simulink model "DataPath"  (R2025a)
settings: Solver=FixedStepAuto  StartTime=0  StopTime=0.02  FixedStep=1e-7  RelTol=1e-3
undefined symbols (not defined in the file): Bit_1, Bit_2, Bit_3, Bit_4, Bit_5, Bit_6, Bit_7, Bit_8
libraries: simulink_extras x126, fl_lib x34, nesl_utility x18, simulink x2
(part 3 of 7)

== system DataPath/Subsystem1/Normalize Div ==
  Enable : Inport
  Step Bus : Inport  Port=2
  MSB : Inport  Port=3
  Eval-ICS : Inport  Port=4
  Store B1-ICS : Inport  Port=5
  Zero : Inport  Port=6
  AND{2..8,10..11} (9 alike) : Logic  IconShape=distinctive  AllPortsSameDT=off  OutDataTypeStr=boolean
  D Latch : simulink_extras/Flip Flops/D Latch
  Demux : Demux  Outputs=5
  OR{,5..7} (4 alike) : Logic  Operator=OR  IconShape=distinctive  AllPortsSameDT=off  OutDataTypeStr=boolean
  S-R Flip-Flop1 : simulink_extras/Flip Flops/S-R Flip-Flop  initial_condition=0
  S-R Flip-Flop2 : simulink_extras/Flip Flops/S-R Flip-Flop  initial_condition=0
  Subsystem1 : Subsystem
  Subsystem8 : Subsystem
  Out ALU : Outport
  Out A1 : Outport  Port=2
  Out B1 : Outport  Port=3
  Store A1 : Outport  Port=4
  Store B1 : Outport  Port=5
  NegA : Outport  Port=6
  ADD : Outport  Port=7
  MSB x : Outport  Port=8
  MSB y : Outport  Port=9
  END-ND : Outport  Port=10
  Div/0 : Outport  Port=11
  wires:
  S-R Flip-Flop1/1 -> AND7/2, OR5/1
  Enable/1 -> AND6/1, AND5/1, AND4/1, AND3/1, AND2/1
  AND2/1 -> OR6/1, D Latch/2
  Subsystem8/2(Q) -> MSB x/1, AND7/1
  S-R Flip-Flop2/1 -> OR6/2, AND8/2, OR5/2
  Subsystem1/2(Q) -> MSB y/1, AND8/1
  AND3/1 -> AND11/1, AND10/1
  AND10/1 -> Div/0/1
  AND5/1 -> S-R Flip-Flop2/1
  MSB/1 -> Subsystem1/1(Data), Subsystem8/1(Data)
  D Latch/2 -> AND11/2
  AND6/1 -> OR7/2, S-R Flip-Flop2/2, END-ND/1
  AND4/1 -> OR7/1
  D Latch/1 -> AND10/2
  Zero/1 -> D Latch/1
  OR7/1 -> S-R Flip-Flop1/2
  Eval-ICS/1 -> Subsystem1/2(CLK)
  OR5/1 -> Out ALU/1
  Store B1-ICS/1 -> Subsystem8/2(CLK)
  OR6/1 -> OR/2
  AND11/1 -> S-R Flip-Flop1/1
  Step Bus/1 -> Demux/1
  Demux/4 -> AND5/2
  Demux/3 -> AND4/2
  Demux/2 -> AND3/2
  Demux/1 -> AND2/2
  Demux/5 -> AND6/2
  AND7/1 -> Store A1/1, Out A1/1, ADD/1, NegA/1
  AND8/1 -> OR/1, Store B1/1
  OR/1 -> Out B1/1

== system DataPath/Subsystem1/SCS ==
  CLR : Inport
  Multiplying : Inport  Port=2
  Dividing : Inport  Port=3
  Evaluating : Inport  Port=4
  Output DP-Mult : Inport  Port=5
  Output DP-Div : Inport  Port=6
  CLK : Inport  Port=7
  END-CD : Inport  Port=8
  END-ND : Inport  Port=9
  DIV/0 : Inport  Port=10
  AND{,1..4} (5 alike) : Logic  IconShape=distinctive  AllPortsSameDT=off  OutDataTypeStr=boolean
  Delay One Step : Delay  DelayLength=1  SampleTime=1e-6
  Delay One Step1 : Delay  DelayLength=1  SampleTime=1e-6
  Delay One Step{2,4..7} (5 alike) : Delay  DelayLength=1
  OR4 : Logic  Operator=OR  Inputs=3  IconShape=distinctive  AllPortsSameDT=off  OutDataTypeStr=boolean
  OR5 : Logic  Operator=OR  IconShape=distinctive  AllPortsSameDT=off  OutDataTypeStr=boolean
  Rate Transition : RateTransition
  Rate Transition1 : RateTransition
  S-R Flip-Flop : simulink_extras/Flip Flops/S-R Flip-Flop  initial_condition=0
  S-R Flip-Flop1 : simulink_extras/Flip Flops/S-R Flip-Flop  initial_condition=0
  S-R Flip-Flop2 : simulink_extras/Flip Flops/S-R Flip-Flop  initial_condition=0
  Enable Stepper : Outport
  CCLK : Outport  Port=2
  Enable-Mult : Outport  Port=3
  Enable-CD : Outport  Port=4
  Enable-ND : Outport  Port=5
  Enable-SDR : Outport  Port=6
  wires:
  CLR/1 -> S-R Flip-Flop2/2, S-R Flip-Flop1/2, Rate Transition1/1
  Output DP-Div/1 -> OR4/2
  DIV/0/1 -> OR4/3
  Output DP-Mult/1 -> OR4/1
  Multiplying/1 -> AND/2
  Dividing/1 -> AND2/1
  Evaluating/1 -> AND2/2, AND/1
  S-R Flip-Flop2/2 -> AND4/2
  END-ND/1 -> Delay One Step1/1
  END-CD/1 -> Delay One Step/1
  OR4/1 -> Delay One Step7/1
  AND2/1 -> OR5/1, AND3/1
  AND/1 -> OR5/2, Delay One Step5/1
  S-R Flip-Flop1/1 -> AND4/1
  S-R Flip-Flop1/2 -> AND3/2
  CLK/1 -> AND1/1
  S-R Flip-Flop/1 -> Delay One Step6/1
  OR5/1 -> Enable Stepper/1
  AND3/1 -> Delay One Step2/1
  AND4/1 -> Rate Transition/1
  AND1/1 -> CCLK/1
  S-R Flip-Flop2/1 -> Delay One Step4/1
  Delay One Step2/1 -> Enable-ND/1
  Rate Transition/1 -> Enable-CD/1
  Delay One Step4/1 -> Enable-SDR/1
  Delay One Step5/1 -> Enable-Mult/1
  Delay One Step/1 -> S-R Flip-Flop2/1
  Delay One Step1/1 -> S-R Flip-Flop1/1
  Delay One Step6/1 -> AND1/2
  Delay One Step7/1 -> S-R Flip-Flop/2
  Rate Transition1/1 -> S-R Flip-Flop/1

== system DataPath/Subsystem1/Sign Div result ==
  Enable : Inport
  Step Bus : Inport  Port=2
  MOD : Inport  Port=3
  MSB x : Inport  Port=4
  MSB y : Inport  Port=5
  AND{,1..9} (10 alike) : Logic  IconShape=distinctive  AllPortsSameDT=off  OutDataTypeStr=boolean
  Delay : Delay  DelayLength=1  InputProcessing=Columns as channels (frame based)  SampleTime=1e-6
  Delay1 : Delay  DelayLength=1  InputProcessing=Columns as channels (frame based)  SampleTime=1e-6
  Delay2 : Delay  DelayLength=1  InputProcessing=Columns as channels (frame based)  SampleTime=1e-6
  Demux : Demux  Outputs=5
  OR{,1..3,5,9} (6 alike) : Logic  Operator=OR  IconShape=distinctive  AllPortsSameDT=off  OutDataTypeStr=boolean
  S-R Flip-Flop{,1..3} (4 alike) : simulink_extras/Flip Flops/S-R Flip-Flop  initial_condition=0
  XOR : Logic  Operator=XOR  IconShape=distinctive  AllPortsSameDT=off  OutDataTypeStr=boolean
  Out ALU : Outport
  Out A1 : Outport  Port=2
  Out B2 : Outport  Port=3
  Store A1 : Outport  Port=4
  Store B2 : Outport  Port=5
  NegA : Outport  Port=6
  Output DP : Outport  Port=7
  ADD : Outport  Port=8
  wires:
  Enable/1 -> AND6/1, AND5/1, AND4/1, AND3/1, AND2/1
  Step Bus/1 -> Demux/1
  Demux/4 -> S-R Flip-Flop3/2, AND5/2
  Demux/3 -> AND4/2
  Demux/2 -> AND3/2
  Demux/1 -> AND2/2, Delay1/1
  Demux/5 -> AND6/2
  MSB y/1 -> XOR/2
  MSB x/1 -> AND7/1, XOR/1
  AND2/1 -> S-R Flip-Flop/1
  OR9/1 -> S-R Flip-Flop/2
  AND3/1 -> Delay2/1, OR9/1
  AND6/1 -> OR2/2, OR9/2, AND9/1, AND/1, AND8/1
  S-R Flip-Flop/1 -> AND1/2
  XOR/1 -> AND1/1
  OR1/1 -> OR5/1, Out B2/1
  AND1/1 -> OR1/1, Store B2/1
  OR2/1 -> S-R Flip-Flop1/2
  AND4/1 -> S-R Flip-Flop1/1
  AND5/1 -> OR2/1
  S-R Flip-Flop1/1 -> AND7/2
  OR3/1 -> OR5/2, Out A1/1
  AND7/1 -> OR/1, OR3/1, Store A1/1, NegA/1
  S-R Flip-Flop3/1 -> AND8/2
  AND/1 -> OR1/2
  AND8/1 -> OR3/2
  OR5/1 -> Out ALU/1
  AND9/1 -> Output DP/1, OR/2
  S-R Flip-Flop2/1 -> Delay/1
  OR/1 -> ADD/1
  MOD/1 -> S-R Flip-Flop3/1
  S-R Flip-Flop3/2 -> AND/2
  Delay/1 -> AND9/2
  Delay1/1 -> S-R Flip-Flop2/2
  Delay2/1 -> S-R Flip-Flop2/1

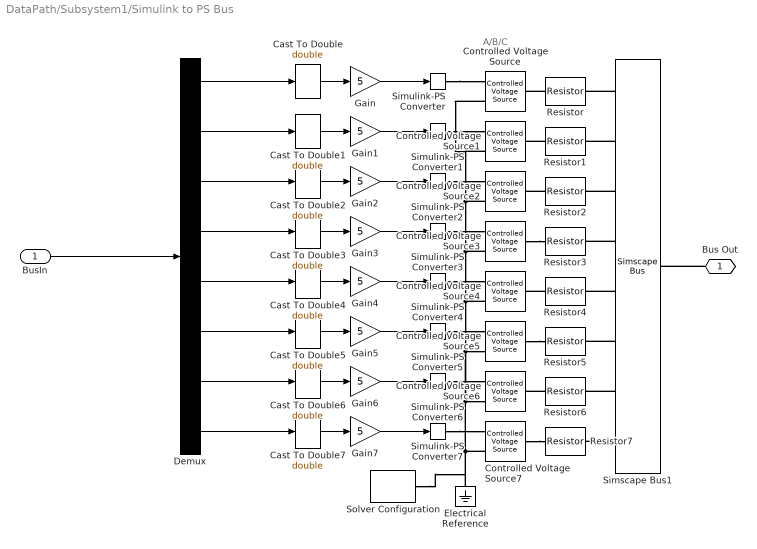
== system DataPath/Subsystem1/Simulink to PS Bus ==
  note: A/B/C
  BusIn : Inport
  Cast To Double{,1..7} (8 alike) : DataTypeConversion  OutDataTypeStr=double  SaturateOnIntegerOverflow=off  RndMeth=Floor
  Controlled Voltage Source{,1..7} (8 alike) : fl_lib/Electrical/Electrical Sources/Controlled Voltage Source
  Demux : Demux  Outputs=8
  Electrical Reference : fl_lib/Electrical/Electrical Elements/Electrical Reference
  Gain{,1..7} (8 alike) : Gain  Gain=5
  Resistor{,1..7} (8 alike) : fl_lib/Electrical/Electrical Elements/Resistor  R=1 Ohm  i_specify=off  i_priority=None  i=0 A  i_nominal_specify=off  i_nominal_value=1  i_nominal_unit=A  v_specify=off  v_priority=None  v=0 V  v_nominal_specify=off  v_nominal_value=1  v_nominal_unit=V
  Simscape Bus1 : SimscapeBus  HierarchyStrings=Bit_8;Bit_7;Bit_6;Bit_5;Bit_4;Bit_3;Bit_2;Bit_1
  Simulink-PS Converter{,1..7} (8 alike) : nesl_utility/Simulink-PS Converter  PhysicalDomain=network_engine_domain  SubClassName=ps_input  LeftPortType=input  RightPortType=output  PseudoPeriodic=off  Frequencies=[]  NoiseDistribution=none  NoiseParameters=[]  Unit=1  AffineConversion=off  FilteringAndDerivatives=provide  SimscapeFilterOrder=1  InputFilterTimeConstant=0.001  UdotUserProvided=0
  Solver Configuration : nesl_utility/Solver Configuration  PhysicalDomain=network_engine_domain  SubClassName=solver  LeftPortType=input  RightPortType=generic  Tones=[]  Harmonics=[]  SimulateNoise=off  Profile=off  UseLocalSampling=off  EnableSwitchedLinearOptims=on  FrequencyDomain=off  UseCCode=off  RelTol=0.001  AbsTol=0.001  MinStep=1e-09  ToWorkspace=off  RevertToSquareIcSolve=off  NumHomotopyIterations=100  PhasorMode=off  PhasorModeNumHarmonics=1  ConsistencySolver=NEWTON_XTOL_AFTER_FTOL  IndexReductionMethod=DerivativeReplacement  DoDC=off  ResidualTolerance=1e-09  ConsistencyTolSource=GLOBAL  ConsistencyAbsTol=0.001  ConsistencyRelTol=0.001  ConsistencyTolFactor=0.001  UseLocalSolver=off  LocalSolverChoice=NE_BACKWARD_EULER_ADVANCER  ResolveIndetEquations=on  FunctionEvalNumThread=1  LocalSolverSampleTime=0.001  DoFixedCost=off  MaxNonlinIter=3  MaxModeIter=2  ComputeImpulses=off  ImpulseIterations=2  LinearAlgebra=auto  LinearAlgebraNumThread=0  EquationFormulation=NE_TIME_EF  DelaysMemoryBudget=1024  AutomaticFiltering=on  FilteringTimeConstant=0.001  PartitionStorageMethod=AS_NEEDED  PartitionMemoryBudget=1024  PartitionMethod=ROBUST  MultibodyUseLocalSolver=off  MultibodyLocalSolverChoice=ODE1  MultibodyLocalSolverSampleTime=0.001
  Bus Out : PMIOPort  Side=Right
  wires:
  BusIn/1 -> Demux/1
  Demux/5 -> Cast To Double4/1
  Cast To Double5/1 -> Gain5/1
  Cast To Double6/1 -> Gain6/1
  Cast To Double7/1 -> Gain7/1
  Gain/1 -> Simulink-PS Converter/1
  Demux/2 -> Cast To Double1/1
  Demux/4 -> Cast To Double3/1
  Gain5/1 -> Simulink-PS Converter5/1
  Gain4/1 -> Simulink-PS Converter4/1
  Gain2/1 -> Simulink-PS Converter2/1
  Cast To Double2/1 -> Gain2/1
  Cast To Double4/1 -> Gain4/1
  Gain6/1 -> Simulink-PS Converter6/1
  Cast To Double3/1 -> Gain3/1
  Cast To Double/1 -> Gain/1
  Cast To Double1/1 -> Gain1/1
  Demux/7 -> Cast To Double6/1
  Demux/1 -> Cast To Double/1
  Gain3/1 -> Simulink-PS Converter3/1
  Demux/6 -> Cast To Double5/1
  Gain7/1 -> Simulink-PS Converter7/1
  Demux/8 -> Cast To Double7/1
  Demux/3 -> Cast To Double2/1
  Gain1/1 -> Simulink-PS Converter1/1
  connections:
  Controlled Voltage Source2/RConn2 -- Controlled Voltage Source/RConn2 -- Controlled Voltage Source1/RConn2 -- Controlled Voltage Source3/RConn2 -- Controlled Voltage Source4/RConn2 -- Controlled Voltage Source5/RConn2 -- Controlled Voltage Source6/RConn2 -- Controlled Voltage Source7/RConn2 -- Solver Configuration/RConn1 -- Electrical Reference/LConn1
  Simscape Bus1/LConn7 -- Resistor6/RConn1
  Simscape Bus1/LConn5 -- Resistor4/RConn1
  Simscape Bus1/LConn8 -- Resistor7/RConn1
  Simulink-PS Converter5/RConn1 -- Controlled Voltage Source5/RConn1
  Simulink-PS Converter4/RConn1 -- Controlled Voltage Source4/RConn1
  Simulink-PS Converter6/RConn1 -- Controlled Voltage Source6/RConn1
  Simulink-PS Converter/RConn1 -- Controlled Voltage Source/RConn1
  Simulink-PS Converter1/RConn1 -- Controlled Voltage Source1/RConn1
  Simscape Bus1/LConn4 -- Resistor3/RConn1
  Controlled Voltage Source5/LConn1 -- Resistor5/LConn1
  Simulink-PS Converter7/RConn1 -- Controlled Voltage Source7/RConn1
  Simulink-PS Converter3/RConn1 -- Controlled Voltage Source3/RConn1
  Simscape Bus1/LConn2 -- Resistor1/RConn1
  Simulink-PS Converter2/RConn1 -- Controlled Voltage Source2/RConn1
  Resistor2/LConn1 -- Controlled Voltage Source2/LConn1
  Resistor/LConn1 -- Controlled Voltage Source/LConn1
  Simscape Bus1/LConn1 -- Resistor/RConn1
  Resistor1/LConn1 -- Controlled Voltage Source1/LConn1
  Simscape Bus1/LConn3 -- Resistor2/RConn1
  Controlled Voltage Source3/LConn1 -- Resistor3/LConn1
  Resistor4/LConn1 -- Controlled Voltage Source4/LConn1
  Simscape Bus1/LConn6 -- Resistor5/RConn1
  Resistor6/LConn1 -- Controlled Voltage Source6/LConn1
  Controlled Voltage Source7/LConn1 -- Resistor7/LConn1
  Bus Out/RConn1 -- Simscape Bus1/RConn1

== system DataPath/Subsystem1/Stepper ==
  Reset : Inport
  Enable : Inport  Port=2
  CLK : Inport  Port=3
  Subsystem1 : Subsystem
      settings: PortSchema="{\"entries\":[{\"content\":{\"sides\":[{\"content\":{\"connectorIds\":[\"In1\",\"Out3\",\"In2\"]},\"type\":\"ConnectorPlacement.EquallySpacedRectSide\",\"uuid\":\"a2ffd4d4-cb1e-427b-87da-e82cfc528a9f\"},{\"content\":{\"connectorIds\":[\"Out1\",\"In3\",\"Out2\"],\"side\":\"RIGHT\"},\"type\":\"ConnectorPlacement.EquallySpacedRectSide\",\"uuid\":\"71314638-bff7-4a07-ab36-c1b86a64e6a5\"},{\"content\":{\"side\":\"TOP\"},\"type\":\"ConnectorPlacement.EquallySpacedRectSide\",\"uuid\":\"4ed90d18-bd24-4652-9ebf-70eb68655746\"},{\"content\":{\"side\":\"BOTTOM\"},\"type\":\"ConnectorPlacement.EquallySpacedRectSide\",\"uuid\":\"b13ca18e-58ec-4b33-9e47-5b828845d5a6\"}]},\"type\":\"ConnectorPlacement.EquallySpacedConnector\",\"uuid\":\"af20c32a-17bf-45dc-90e2-7848574669b1\"}],\"packageUris\":[\"http://schema.mathworks.com/mf0/Connector/R2020b\"],\"version\":\"1.0\"}"
  Subsystem2 : Subsystem
      settings: PortSchema="{\"entries\":[{\"content\":{\"sides\":[{\"content\":{\"connectorIds\":[\"In1\",\"Out3\",\"In2\"]},\"type\":\"ConnectorPlacement.EquallySpacedRectSide\",\"uuid\":\"a2ffd4d4-cb1e-427b-87da-e82cfc528a9f\"},{\"content\":{\"connectorIds\":[\"Out1\",\"In3\",\"Out2\"],\"side\":\"RIGHT\"},\"type\":\"ConnectorPlacement.EquallySpacedRectSide\",\"uuid\":\"71314638-bff7-4a07-ab36-c1b86a64e6a5\"},{\"content\":{\"side\":\"TOP\"},\"type\":\"ConnectorPlacement.EquallySpacedRectSide\",\"uuid\":\"4ed90d18-bd24-4652-9ebf-70eb68655746\"},{\"content\":{\"side\":\"BOTTOM\"},\"type\":\"ConnectorPlacement.EquallySpacedRectSide\",\"uuid\":\"b13ca18e-58ec-4b33-9e47-5b828845d5a6\"}]},\"type\":\"ConnectorPlacement.EquallySpacedConnector\",\"uuid\":\"af20c32a-17bf-45dc-90e2-7848574669b1\"}],\"packageUris\":[\"http://schema.mathworks.com/mf0/Connector/R2020b\"],\"version\":\"1.0\"}"
  Subsystem3 : Subsystem
      settings: PortSchema="{\"entries\":[{\"content\":{\"sides\":[{\"content\":{\"connectorIds\":[\"In1\",\"Out3\",\"In2\"]},\"type\":\"ConnectorPlacement.EquallySpacedRectSide\",\"uuid\":\"a2ffd4d4-cb1e-427b-87da-e82cfc528a9f\"},{\"content\":{\"connectorIds\":[\"Out1\",\"In3\",\"Out2\"],\"side\":\"RIGHT\"},\"type\":\"ConnectorPlacement.EquallySpacedRectSide\",\"uuid\":\"71314638-bff7-4a07-ab36-c1b86a64e6a5\"},{\"content\":{\"side\":\"TOP\"},\"type\":\"ConnectorPlacement.EquallySpacedRectSide\",\"uuid\":\"4ed90d18-bd24-4652-9ebf-70eb68655746\"},{\"content\":{\"side\":\"BOTTOM\"},\"type\":\"ConnectorPlacement.EquallySpacedRectSide\",\"uuid\":\"b13ca18e-58ec-4b33-9e47-5b828845d5a6\"}]},\"type\":\"ConnectorPlacement.EquallySpacedConnector\",\"uuid\":\"af20c32a-17bf-45dc-90e2-7848574669b1\"}],\"packageUris\":[\"http://schema.mathworks.com/mf0/Connector/R2020b\"],\"version\":\"1.0\"}"
  Subsystem4 : Subsystem
      settings: PortSchema="{\"entries\":[{\"content\":{\"sides\":[{\"content\":{\"connectorIds\":[\"In1\",\"Out3\",\"In2\"]},\"type\":\"ConnectorPlacement.EquallySpacedRectSide\",\"uuid\":\"a2ffd4d4-cb1e-427b-87da-e82cfc528a9f\"},{\"content\":{\"connectorIds\":[\"Out1\",\"In3\",\"Out2\"],\"side\":\"RIGHT\"},\"type\":\"ConnectorPlacement.EquallySpacedRectSide\",\"uuid\":\"71314638-bff7-4a07-ab36-c1b86a64e6a5\"},{\"content\":{\"side\":\"TOP\"},\"type\":\"ConnectorPlacement.EquallySpacedRectSide\",\"uuid\":\"4ed90d18-bd24-4652-9ebf-70eb68655746\"},{\"content\":{\"side\":\"BOTTOM\"},\"type\":\"ConnectorPlacement.EquallySpacedRectSide\",\"uuid\":\"b13ca18e-58ec-4b33-9e47-5b828845d5a6\"}]},\"type\":\"ConnectorPlacement.EquallySpacedConnector\",\"uuid\":\"af20c32a-17bf-45dc-90e2-7848574669b1\"}],\"packageUris\":[\"http://schema.mathworks.com/mf0/Connector/R2020b\"],\"version\":\"1.0\"}"
  Step 0 : Outport
  Step 1 : Outport  Port=2
  Step 2 : Outport  Port=3
  Step 3 : Outport  Port=4
  Step 4 : Outport  Port=5
  wires:
  CLK/1 -> Subsystem1/2(CLK), Subsystem4/2(CLK), Subsystem3/2(CLK), Subsystem2/2(CLK)
  Subsystem4/1("Step_{n}") -> Step 4/1
  Reset/1 -> Subsystem4/3("OR_{n+1}")
  Enable/1 -> Subsystem2/1("Step_{n-1}")
  Subsystem2/1("Step_{n}") -> Subsystem1/1("Step_{n-1}"), Step 1/1
  Subsystem1/3("OR_{n}") -> Subsystem2/3("OR_{n+1}")
  Subsystem1/1("Step_{n}") -> Subsystem3/1("Step_{n-1}"), Step 2/1
  Subsystem3/3("OR_{n}") -> Subsystem1/3("OR_{n+1}")
  Subsystem3/1("Step_{n}") -> Subsystem4/1("Step_{n-1}"), Step 3/1
  Subsystem4/3("OR_{n}") -> Subsystem3/3("OR_{n+1}")
  Subsystem2/2("!Step_{n}") -> Step 0/1

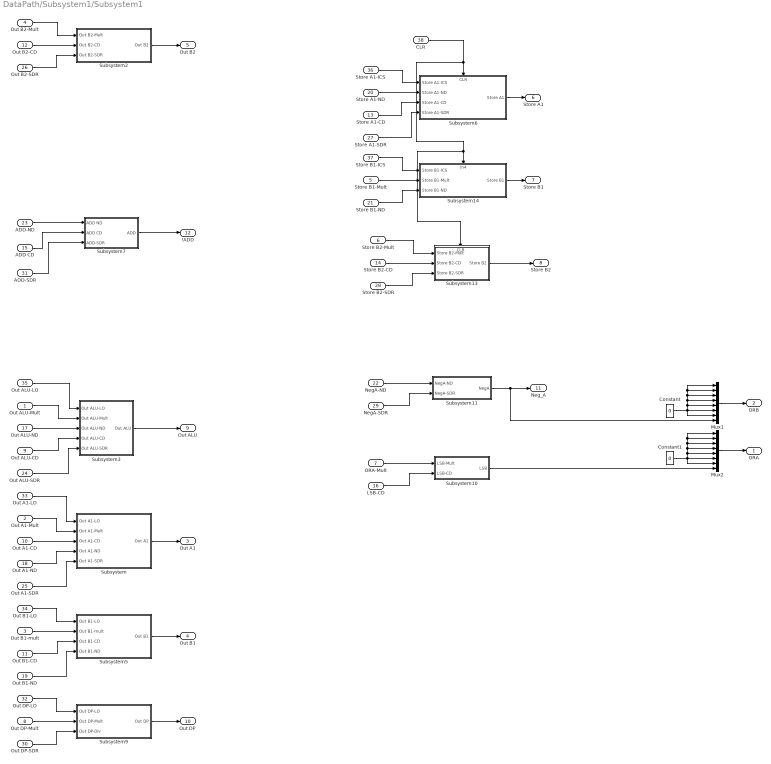
== system DataPath/Subsystem1/Subsystem1 ==
  Out ALU-Mult : Inport
  Out A1-Mult : Inport  Port=2
  Out B1-mult : Inport  Port=3
  Out B2-Mult : Inport  Port=4
  Store B1-Mult : Inport  Port=5
  Store B2-Mult : Inport  Port=6
  ORA-Mult : Inport  Port=7
  Out DP-Mult : Inport  Port=8
  Out ALU-CD : Inport  Port=9
  Out A1-CD : Inport  Port=10
  Out B1-CD : Inport  Port=11
  Out B2-CD : Inport  Port=12
  Store A1-CD : Inport  Port=13
  Store B2-CD : Inport  Port=14
  ADD CD : Inport  Port=15
  LSB-CD : Inport  Port=16
  Out ALU-ND : Inport  Port=17
  Out A1-ND : Inport  Port=18
  Out B1-ND : Inport  Port=19
  Store A1-ND : Inport  Port=20
  Store B1-ND : Inport  Port=21
  NegA-ND : Inport  Port=22
  ADD-ND : Inport  Port=23
  Out ALU-SDR : Inport  Port=24
  Out A1-SDR : Inport  Port=25
  Out B2-SDR : Inport  Port=26
  Store A1-SDR : Inport  Port=27
  Store B2-SDR : Inport  Port=28
  NegA-SDR : Inport  Port=29
  Out DP-SDR : Inport  Port=30
  ADD-SDR : Inport  Port=31
  Out DP-LO : Inport  Port=32
  Out A1-LO : Inport  Port=33
  Out B1-LO : Inport  Port=34
  Out ALU-LO : Inport  Port=35
  Store A1-ICS : Inport  Port=36
  Store B1-ICS : Inport  Port=37
  CLR : Inport  Port=38
  Constant : Constant  Value=0  OutDataTypeStr=boolean
  Constant1 : Constant  Value=0  OutDataTypeStr=boolean
  Mux1 : Mux  Inputs=8
  Mux2 : Mux  Inputs=8
  Subsystem : Subsystem
  Subsystem10 : Subsystem
  Subsystem11 : Subsystem
  Subsystem13 : Subsystem
      settings: PortSchema="{\"entries\":[{\"content\":{\"sides\":[{\"content\":{\"connectorIds\":[\"In1\",\"In2\",\"In3\"]},\"type\":\"ConnectorPlacement.EquallySpacedRectSide\",\"uuid\":\"2d56d23b-6617-4046-a99f-24fef166ef06\"},{\"content\":{\"connectorIds\":[\"Out1\"],\"side\":\"RIGHT\"},\"type\":\"ConnectorPlacement.EquallySpacedRectSide\",\"uuid\":\"3c4df583-b380-4f6c-803a-8385e40aa290\"},{\"content\":{\"connectorIds\":[\"In4\"],\"side\":\"TOP\"},\"type\":\"ConnectorPlacement.EquallySpacedRectSide\",\"uuid\":\"43dc231e-5ab9-4cdd-8239-1dcaab484e6e\"}]},\"type\":\"ConnectorPlacement.EquallySpacedConnector\",\"uuid\":\"3f11ba61-6682-48c0-a60b-53ec54e9a9d7\"}],\"packageUris\":[\"http://schema.mathworks.com/mf0/Connector/R2020b\"],\"version\":\"1.0\"}"
  Subsystem14 : Subsystem
      settings: PortSchema="{\"entries\":[{\"content\":{\"sides\":[{\"content\":{\"connectorIds\":[\"In1\",\"In2\",\"In3\"]},\"type\":\"ConnectorPlacement.EquallySpacedRectSide\",\"uuid\":\"2d56d23b-6617-4046-a99f-24fef166ef06\"},{\"content\":{\"connectorIds\":[\"Out1\"],\"side\":\"RIGHT\"},\"type\":\"ConnectorPlacement.EquallySpacedRectSide\",\"uuid\":\"3c4df583-b380-4f6c-803a-8385e40aa290\"},{\"content\":{\"connectorIds\":[\"In4\"],\"side\":\"TOP\"},\"type\":\"ConnectorPlacement.EquallySpacedRectSide\",\"uuid\":\"43dc231e-5ab9-4cdd-8239-1dcaab484e6e\"}]},\"type\":\"ConnectorPlacement.EquallySpacedConnector\",\"uuid\":\"3f11ba61-6682-48c0-a60b-53ec54e9a9d7\"}],\"packageUris\":[\"http://schema.mathworks.com/mf0/Connector/R2020b\"],\"version\":\"1.0\"}"
  Subsystem2 : Subsystem
  Subsystem3 : Subsystem
  Subsystem5 : Subsystem
  Subsystem6 : Subsystem
      settings: PortSchema="{\"entries\":[{\"content\":{\"sides\":[{\"content\":{\"connectorIds\":[\"In1\",\"In2\",\"In3\",\"In4\"]},\"type\":\"ConnectorPlacement.EquallySpacedRectSide\",\"uuid\":\"1cc443aa-38b6-479c-9624-02afc8875fe2\"},{\"content\":{\"connectorIds\":[\"Out1\"],\"side\":\"RIGHT\"},\"type\":\"ConnectorPlacement.EquallySpacedRectSide\",\"uuid\":\"f78e015e-8990-42cd-9709-a04196c9d570\"},{\"content\":{\"connectorIds\":[\"In5\"],\"side\":\"TOP\"},\"type\":\"ConnectorPlacement.EquallySpacedRectSide\",\"uuid\":\"6baf1ba9-0262-41fa-84ed-1502284065d7\"}]},\"type\":\"ConnectorPlacement.EquallySpacedConnector\",\"uuid\":\"f889b3e3-665a-4999-a847-f3de4112163d\"}],\"packageUris\":[\"http://schema.mathworks.com/mf0/Connector/R2020b\"],\"version\":\"1.0\"}"
  Subsystem7 : Subsystem
  Subsystem9 : Subsystem
  ORA : Outport
  ORB : Outport  Port=2
  Out A1 : Outport  Port=3
  Out B1 : Outport  Port=4
  Out B2 : Outport  Port=5
  Store A1 : Outport  Port=6
  Store B1 : Outport  Port=7
  Store B2 : Outport  Port=8
  Out ALU : Outport  Port=9
  Out DP : Outport  Port=10
  Neg_A : Outport  Port=11
  "!ADD " : Outport  Port=12
  wires:
  Subsystem7/1("ADD ") -> "!ADD "/1
  Out B2-CD/1 -> Subsystem2/2(Out B2-CD)
  Store A1-CD/1 -> Subsystem6/3(Store A1-CD)
  Store B1-ICS/1 -> Subsystem14/1(Store B1-ICS)
  Store A1-ICS/1 -> Subsystem6/1(Store A1-ICS)
  Out B1-mult/1 -> Subsystem5/2(Out B1-mult)
  Out B2-Mult/1 -> Subsystem2/1(Out B2-Mult)
  Out A1-SDR/1 -> Subsystem/5(Out A1-SDR)
  Out B2-SDR/1 -> Subsystem2/3(Out B2-SDR)
  Out ALU-SDR/1 -> Subsystem3/5(Out ALU-SDR)
  LSB-CD/1 -> Subsystem10/2(LSB-CD)
  Out DP-Mult/1 -> Subsystem9/2(Out DP-Mult)
  ORA-Mult/1 -> Subsystem10/1(LSB-Mult)
  Out B1-CD/1 -> Subsystem5/3(Out B1-CD)
  Store A1-ND/1 -> Subsystem6/2(Store A1-ND)
  Subsystem9/1(Out DP) -> Out DP/1
  Store B2-SDR/1 -> Subsystem13/3(Store B2-SDR)
  Store A1-SDR/1 -> Subsystem6/4(Store A1-SDR)
  Store B1-ND/1 -> Subsystem14/3(Store B1-ND)
  ADD-ND/1 -> Subsystem7/1(ADD ND)
  Store B2-CD/1 -> Subsystem13/2(Store B2-CD)
  ADD CD/1 -> Subsystem7/2(ADD CD)
  Out ALU-CD/1 -> Subsystem3/4(Out ALU-CD)
  NegA-ND/1 -> Subsystem11/1(NegA-ND)
  Out DP-SDR/1 -> Subsystem9/3(Out DP-Div)
  NegA-SDR/1 -> Subsystem11/2(NegA-SDR)
  Subsystem6/1(Store A1) -> Store A1/1
  Store B2-Mult/1 -> Subsystem13/1(Store B2-Mult)
  Store B1-Mult/1 -> Subsystem14/2(Store B1-Mult)
  Out B1-LO/1 -> Subsystem5/1(Out B1-LO)
  Out ALU-LO/1 -> Subsystem3/1(Out ALU-LO)
  Out A1-Mult/1 -> Subsystem/2(Out A1-Mult)
  Out ALU-Mult/1 -> Subsystem3/2(Out ALU-Mult)
  Out A1-CD/1 -> Subsystem/3(Out A1-CD)
  Out ALU-ND/1 -> Subsystem3/3(Out ALU-ND)
  Out DP-LO/1 -> Subsystem9/1(Out DP-LO)
  Out A1-LO/1 -> Subsystem/1(Out A1-LO)
  Out B1-ND/1 -> Subsystem5/4(Out B1-ND)
  Out A1-ND/1 -> Subsystem/4(Out A1-ND)
  Subsystem2/1(Out B2) -> Out B2/1
  Subsystem14/1(Store B1) -> Store B1/1
  Subsystem3/1(Out ALU) -> Out ALU/1
  Subsystem/1(Out A1) -> Out A1/1
  Subsystem5/1(Out B1) -> Out B1/1
  Subsystem13/1(Store B2) -> Store B2/1
  CLR/1 -> Subsystem13/4(CLR), Subsystem14/4(In4), Subsystem6/5(CLR)
  Subsystem11/1(NegA) -> Mux1/8, Neg_A/1
  Mux1/1 -> ORB/1
  Constant/1 -> Mux1/7, Mux1/1, Mux1/2, Mux1/3, Mux1/4, Mux1/5, Mux1/6
  Mux2/1 -> ORA/1
  Subsystem10/1(LSB) -> Mux2/8
  Constant1/1 -> Mux2/7, Mux2/1, Mux2/2, Mux2/3, Mux2/4, Mux2/5, Mux2/6
  ADD-SDR/1 -> Subsystem7/3(ADD-SDR)

== system DataPath/Subsystem1/Subsystem4 ==
  Output ALU : Inport
  Enable Main Input : Inport  Port=2
  ALU Bus : Inport  Port=3
  Main Input : Inport  Port=4
  Cast To Boolean : DataTypeConversion  OutDataTypeStr=boolean  SaturateOnIntegerOverflow=off  RndMeth=Floor
  Delay One Step1 : Delay  DelayLength=1
  Delay One Step4 : Delay  DelayLength=1
  Demux : Demux  Outputs=8
  Demux1 : Demux  Outputs=8
  MATLAB Function : MATLAB Function  TreatAsAtomicUnit=on
  Multiport Switch{1..4,6..9} (8 alike) : MultiPortSwitch  DataPortOrder=Specify indices  DataPortIndices={0,1,2,-1}  SaturateOnIntegerOverflow=off  InputSameDT=off
  Mux : Mux  Inputs=8
  Zero{1..8} (8 alike) : Constant  Value=0  OutDataTypeStr=Inherit: Inherit via back propagation
  MSB : Outport
  DP Bus : Outport  Port=2
  wires:
  ALU Bus/1 -> Delay One Step4/1
  Main Input/1 -> Delay One Step1/1
  Mux/1 -> DP Bus/1
  Enable Main Input/1 -> MATLAB Function/1(MainInput)
  Zero8/1 -> Multiport Switch8/5
  Zero1/1 -> Multiport Switch1/5
  Zero3/1 -> Multiport Switch2/5
  Zero2/1 -> Multiport Switch3/5
  Zero4/1 -> Multiport Switch6/5
  Zero5/1 -> Multiport Switch4/5
  Zero6/1 -> Multiport Switch9/5
  Zero7/1 -> Multiport Switch7/5
  MATLAB Function/1(Select) -> Multiport Switch8/1, Multiport Switch1/1, Multiport Switch2/1, Multiport Switch3/1, Multiport Switch4/1, Multiport Switch6/1, Multiport Switch7/1, Multiport Switch9/1
  Demux1/1 -> Multiport Switch8/3
  Demux1/2 -> Multiport Switch1/3
  Demux1/3 -> Multiport Switch2/3
  Demux1/4 -> Multiport Switch3/3
  Demux1/5 -> Multiport Switch4/3
  Demux1/6 -> Multiport Switch6/3
  Demux1/7 -> Multiport Switch7/3
  Demux1/8 -> Multiport Switch9/3
  Multiport Switch8/1 -> MSB/1, Mux/1
  Multiport Switch9/1 -> Mux/8
  Multiport Switch7/1 -> Mux/7
  Multiport Switch6/1 -> Mux/6
  Multiport Switch4/1 -> Mux/5
  Multiport Switch3/1 -> Mux/4
  Multiport Switch1/1 -> Mux/2
  Multiport Switch2/1 -> Mux/3
  Output ALU/1 -> MATLAB Function/2(ALU)
  Cast To Boolean/1 -> Demux/1
  Delay One Step4/1 -> Demux1/1
  Delay One Step1/1 -> Cast To Boolean/1
  Demux/1 -> Multiport Switch8/2
  Demux/2 -> Multiport Switch1/2
  Demux/3 -> Multiport Switch2/2
  Demux/4 -> Multiport Switch3/2
  Demux/5 -> Multiport Switch4/2
  Demux/6 -> Multiport Switch6/2
  Demux/7 -> Multiport Switch7/2
  Demux/8 -> Multiport Switch9/2

== system DataPath/Subsystem/ALU/ALU MUX ==
  note: Each Enabler is a set of 8 tri-state buffers
  0/0/0 : Inport
  0/0/1 : Inport  Port=2
  0/1/0 : Inport  Port=3
  0/1/1 : Inport  Port=4
  1/0/0 : Inport  Port=5
  1/0/1 : Inport  Port=6
  1/1/0 : Inport  Port=7
  1/1/1 : Inport  Port=8
  Bus1 : Inport  Port=9
  Bus2 : Inport  Port=10
  Bus3 : Inport  Port=11
  Bus4 : Inport  Port=12
  Bus5 : Inport  Port=13
  Bus6 : Inport  Port=14
  Bus7 : Inport  Port=15
  Bus8 : Inport  Port=16
  Delay One Step1 : Delay  DelayLength=1
  Delay One Step3 : Delay  DelayLength=1
  MATLAB Function1 : MATLAB Function  TreatAsAtomicUnit=on
  MATLAB Function2 : MATLAB Function  TreatAsAtomicUnit=on
  MATLAB Function3 : MATLAB Function  TreatAsAtomicUnit=on
  MATLAB Function4 : MATLAB Function  TreatAsAtomicUnit=on
  MATLAB Function5 : MATLAB Function  TreatAsAtomicUnit=on
  MATLAB Function6 : MATLAB Function  TreatAsAtomicUnit=on
  MATLAB Function7 : MATLAB Function  TreatAsAtomicUnit=on
  MATLAB Function8 : MATLAB Function  TreatAsAtomicUnit=on
  Mux : Mux  Inputs=8
  Mux1 : Mux  Inputs=8
  ALU Output : Outport
  wires:
  1/1/1/1 -> Mux/8
  1/1/0/1 -> Mux/7
  1/0/1/1 -> Mux/6
  1/0/0/1 -> Mux/5
  0/1/1/1 -> Mux/4
  0/1/0/1 -> Mux/3
  0/0/1/1 -> Mux/2
  0/0/0/1 -> Mux/1
  Bus3/1 -> MATLAB Function2/1(InputBus)
  Bus5/1 -> MATLAB Function4/1(InputBus)
  Bus8/1 -> MATLAB Function8/1(InputBus)
  Bus2/1 -> MATLAB Function6/1(InputBus)
  Bus4/1 -> MATLAB Function3/1(InputBus)
  Bus1/1 -> MATLAB Function1/1(InputBus)
  Bus6/1 -> MATLAB Function5/1(InputBus)
  Bus7/1 -> MATLAB Function7/1(InputBus)
  Mux/1 -> MATLAB Function8/2(Selection), MATLAB Function7/2(Selection), MATLAB Function5/2(Selection), MATLAB Function4/2(Selection), MATLAB Function3/2(Selection), MATLAB Function2/2(Selection), MATLAB Function1/2(Selection), MATLAB Function6/2(Selection)
  MATLAB Function6/1(output) -> Mux1/2
  MATLAB Function2/1(output) -> Mux1/3
  MATLAB Function3/1(output) -> Mux1/4
  MATLAB Function4/1(output) -> Mux1/5
  MATLAB Function5/1(output) -> Mux1/6
  MATLAB Function7/1(output) -> Mux1/7
  MATLAB Function8/1(output) -> Mux1/8
  MATLAB Function1/1(output) -> Mux1/1
  Mux1/1 -> Delay One Step1/1
  Delay One Step1/1 -> ALU Output/1

== system DataPath/Subsystem/ALU/Adder & Logic Module ==
  Subtract mode : Inport
  Neg_A : Inport  Port=2
  Bus_A : Inport  Port=3
  Bus_B : Inport  Port=4
  Constant : Constant
  Constant1 : Constant  Value=0
  Delay One Step1 : Delay  DelayLength=1
  Delay One Step3 : Delay  DelayLength=1
  Demux1 : Demux  Outputs=8
  Demux2 : Demux  Outputs=8
  Display1 : Display
  Display3 : Display
  MATLAB Function1 : MATLAB Function  TreatAsAtomicUnit=on
  MATLAB Function3 : MATLAB Function  TreatAsAtomicUnit=on
  Subsystem1 : Subsystem
      settings: PortSchema="{\"entries\":[{\"content\":{\"sides\":[{\"content\":{\"connectorIds\":[\"In1\",\"In2\",\"Out3\",\"Out4\"]},\"type\":\"ConnectorPlacement.EquallySpacedRectSide\",\"uuid\":\"d566efe6-1fc5-4e96-a6c3-64a47f89d9c9\"},{\"content\":{\"connectorIds\":[\"Out1\",\"In6\",\"In7\"],\"side\":\"RIGHT\"},\"type\":\"ConnectorPlacement.EquallySpacedRectSide\",\"uuid\":\"006cd780-973d-4bae-abc8-89f745b28566\"},{\"content\":{\"connectorIds\":[\"In3\",\"In4\"],\"side\":\"TOP\"},\"type\":\"ConnectorPlacement.EquallySpacedRectSide\",\"uuid\":\"c760ecb1-3a5c-4ba0-9224-1c9b5ce710fd\"},{\"content\":{\"connectorIds\":[\"In5\",\"Out2\"],\"side\":\"BOTTOM\"},\"type\":\"ConnectorPlacement.EquallySpacedRectSide\",\"uuid\":\"178f6c5d-529f-4f0d-80ca-fb6729cf398e\"}]},\"type\":\"ConnectorPlacement.EquallySpacedConnector\",\"uuid\":\"d5293939-72db-46a2-88f3-163e4f70d202\"}],\"packageUris\":[\"http://schema.mathworks.com/mf0/Connector/R2020b\"],\"version\":\"1.0\"}"
  Subsystem2 : Subsystem
      settings: PortSchema="{\"entries\":[{\"content\":{\"sides\":[{\"content\":{\"connectorIds\":[\"In1\",\"In2\",\"Out3\",\"Out4\"]},\"type\":\"ConnectorPlacement.EquallySpacedRectSide\",\"uuid\":\"d566efe6-1fc5-4e96-a6c3-64a47f89d9c9\"},{\"content\":{\"connectorIds\":[\"Out1\",\"In6\",\"In7\"],\"side\":\"RIGHT\"},\"type\":\"ConnectorPlacement.EquallySpacedRectSide\",\"uuid\":\"006cd780-973d-4bae-abc8-89f745b28566\"},{\"content\":{\"connectorIds\":[\"In3\",\"In4\"],\"side\":\"TOP\"},\"type\":\"ConnectorPlacement.EquallySpacedRectSide\",\"uuid\":\"c760ecb1-3a5c-4ba0-9224-1c9b5ce710fd\"},{\"content\":{\"connectorIds\":[\"In5\",\"Out2\"],\"side\":\"BOTTOM\"},\"type\":\"ConnectorPlacement.EquallySpacedRectSide\",\"uuid\":\"178f6c5d-529f-4f0d-80ca-fb6729cf398e\"}]},\"type\":\"ConnectorPlacement.EquallySpacedConnector\",\"uuid\":\"d5293939-72db-46a2-88f3-163e4f70d202\"}],\"packageUris\":[\"http://schema.mathworks.com/mf0/Connector/R2020b\"],\"version\":\"1.0\"}"
  Subsystem3 : Subsystem
      settings: PortSchema="{\"entries\":[{\"content\":{\"sides\":[{\"content\":{\"connectorIds\":[\"In1\",\"In2\",\"Out3\",\"Out4\"]},\"type\":\"ConnectorPlacement.EquallySpacedRectSide\",\"uuid\":\"d566efe6-1fc5-4e96-a6c3-64a47f89d9c9\"},{\"content\":{\"connectorIds\":[\"Out1\",\"In6\",\"In7\"],\"side\":\"RIGHT\"},\"type\":\"ConnectorPlacement.EquallySpacedRectSide\",\"uuid\":\"006cd780-973d-4bae-abc8-89f745b28566\"},{\"content\":{\"connectorIds\":[\"In3\",\"In4\"],\"side\":\"TOP\"},\"type\":\"ConnectorPlacement.EquallySpacedRectSide\",\"uuid\":\"c760ecb1-3a5c-4ba0-9224-1c9b5ce710fd\"},{\"content\":{\"connectorIds\":[\"In5\",\"Out2\"],\"side\":\"BOTTOM\"},\"type\":\"ConnectorPlacement.EquallySpacedRectSide\",\"uuid\":\"178f6c5d-529f-4f0d-80ca-fb6729cf398e\"}]},\"type\":\"ConnectorPlacement.EquallySpacedConnector\",\"uuid\":\"d5293939-72db-46a2-88f3-163e4f70d202\"}],\"packageUris\":[\"http://schema.mathworks.com/mf0/Connector/R2020b\"],\"version\":\"1.0\"}"
  Subsystem4 : Subsystem
      settings: PortSchema="{\"entries\":[{\"content\":{\"sides\":[{\"content\":{\"connectorIds\":[\"In1\",\"In2\",\"Out3\",\"Out4\"]},\"type\":\"ConnectorPlacement.EquallySpacedRectSide\",\"uuid\":\"d566efe6-1fc5-4e96-a6c3-64a47f89d9c9\"},{\"content\":{\"connectorIds\":[\"Out1\",\"In6\",\"In7\"],\"side\":\"RIGHT\"},\"type\":\"ConnectorPlacement.EquallySpacedRectSide\",\"uuid\":\"006cd780-973d-4bae-abc8-89f745b28566\"},{\"content\":{\"connectorIds\":[\"In3\",\"In4\"],\"side\":\"TOP\"},\"type\":\"ConnectorPlacement.EquallySpacedRectSide\",\"uuid\":\"c760ecb1-3a5c-4ba0-9224-1c9b5ce710fd\"},{\"content\":{\"connectorIds\":[\"In5\",\"Out2\"],\"side\":\"BOTTOM\"},\"type\":\"ConnectorPlacement.EquallySpacedRectSide\",\"uuid\":\"178f6c5d-529f-4f0d-80ca-fb6729cf398e\"}]},\"type\":\"ConnectorPlacement.EquallySpacedConnector\",\"uuid\":\"d5293939-72db-46a2-88f3-163e4f70d202\"}],\"packageUris\":[\"http://schema.mathworks.com/mf0/Connector/R2020b\"],\"version\":\"1.0\"}"
  Subsystem5 : Subsystem
      settings: PortSchema="{\"entries\":[{\"content\":{\"sides\":[{\"content\":{\"connectorIds\":[\"In1\",\"In2\",\"Out3\",\"Out4\"]},\"type\":\"ConnectorPlacement.EquallySpacedRectSide\",\"uuid\":\"d566efe6-1fc5-4e96-a6c3-64a47f89d9c9\"},{\"content\":{\"connectorIds\":[\"Out1\",\"In6\",\"In7\"],\"side\":\"RIGHT\"},\"type\":\"ConnectorPlacement.EquallySpacedRectSide\",\"uuid\":\"006cd780-973d-4bae-abc8-89f745b28566\"},{\"content\":{\"connectorIds\":[\"In3\",\"In4\"],\"side\":\"TOP\"},\"type\":\"ConnectorPlacement.EquallySpacedRectSide\",\"uuid\":\"c760ecb1-3a5c-4ba0-9224-1c9b5ce710fd\"},{\"content\":{\"connectorIds\":[\"In5\",\"Out2\"],\"side\":\"BOTTOM\"},\"type\":\"ConnectorPlacement.EquallySpacedRectSide\",\"uuid\":\"178f6c5d-529f-4f0d-80ca-fb6729cf398e\"}]},\"type\":\"ConnectorPlacement.EquallySpacedConnector\",\"uuid\":\"d5293939-72db-46a2-88f3-163e4f70d202\"}],\"packageUris\":[\"http://schema.mathworks.com/mf0/Connector/R2020b\"],\"version\":\"1.0\"}"
  Subsystem6 : Subsystem
      settings: PortSchema="{\"entries\":[{\"content\":{\"sides\":[{\"content\":{\"connectorIds\":[\"In1\",\"In2\",\"Out3\",\"Out4\"]},\"type\":\"ConnectorPlacement.EquallySpacedRectSide\",\"uuid\":\"d566efe6-1fc5-4e96-a6c3-64a47f89d9c9\"},{\"content\":{\"connectorIds\":[\"Out1\",\"In6\",\"In7\"],\"side\":\"RIGHT\"},\"type\":\"ConnectorPlacement.EquallySpacedRectSide\",\"uuid\":\"006cd780-973d-4bae-abc8-89f745b28566\"},{\"content\":{\"connectorIds\":[\"In3\",\"In4\"],\"side\":\"TOP\"},\"type\":\"ConnectorPlacement.EquallySpacedRectSide\",\"uuid\":\"c760ecb1-3a5c-4ba0-9224-1c9b5ce710fd\"},{\"content\":{\"connectorIds\":[\"In5\",\"Out2\"],\"side\":\"BOTTOM\"},\"type\":\"ConnectorPlacement.EquallySpacedRectSide\",\"uuid\":\"178f6c5d-529f-4f0d-80ca-fb6729cf398e\"}]},\"type\":\"ConnectorPlacement.EquallySpacedConnector\",\"uuid\":\"d5293939-72db-46a2-88f3-163e4f70d202\"}],\"packageUris\":[\"http://schema.mathworks.com/mf0/Connector/R2020b\"],\"version\":\"1.0\"}"
  Subsystem7 : Subsystem
      settings: PortSchema="{\"entries\":[{\"content\":{\"sides\":[{\"content\":{\"connectorIds\":[\"In1\",\"In2\",\"Out3\",\"Out4\"]},\"type\":\"ConnectorPlacement.EquallySpacedRectSide\",\"uuid\":\"d566efe6-1fc5-4e96-a6c3-64a47f89d9c9\"},{\"content\":{\"connectorIds\":[\"Out1\",\"In6\",\"In7\"],\"side\":\"RIGHT\"},\"type\":\"ConnectorPlacement.EquallySpacedRectSide\",\"uuid\":\"006cd780-973d-4bae-abc8-89f745b28566\"},{\"content\":{\"connectorIds\":[\"In3\",\"In4\"],\"side\":\"TOP\"},\"type\":\"ConnectorPlacement.EquallySpacedRectSide\",\"uuid\":\"c760ecb1-3a5c-4ba0-9224-1c9b5ce710fd\"},{\"content\":{\"connectorIds\":[\"In5\",\"Out2\"],\"side\":\"BOTTOM\"},\"type\":\"ConnectorPlacement.EquallySpacedRectSide\",\"uuid\":\"178f6c5d-529f-4f0d-80ca-fb6729cf398e\"}]},\"type\":\"ConnectorPlacement.EquallySpacedConnector\",\"uuid\":\"d5293939-72db-46a2-88f3-163e4f70d202\"}],\"packageUris\":[\"http://schema.mathworks.com/mf0/Connector/R2020b\"],\"version\":\"1.0\"}"
  Subsystem8 : Subsystem
      settings: PortSchema="{\"entries\":[{\"content\":{\"sides\":[{\"content\":{\"connectorIds\":[\"In1\",\"In2\",\"Out3\",\"Out4\"]},\"type\":\"ConnectorPlacement.EquallySpacedRectSide\",\"uuid\":\"d566efe6-1fc5-4e96-a6c3-64a47f89d9c9\"},{\"content\":{\"connectorIds\":[\"Out1\",\"In6\",\"In7\"],\"side\":\"RIGHT\"},\"type\":\"ConnectorPlacement.EquallySpacedRectSide\",\"uuid\":\"006cd780-973d-4bae-abc8-89f745b28566\"},{\"content\":{\"connectorIds\":[\"In3\",\"In4\"],\"side\":\"TOP\"},\"type\":\"ConnectorPlacement.EquallySpacedRectSide\",\"uuid\":\"c760ecb1-3a5c-4ba0-9224-1c9b5ce710fd\"},{\"content\":{\"connectorIds\":[\"In5\",\"Out2\"],\"side\":\"BOTTOM\"},\"type\":\"ConnectorPlacement.EquallySpacedRectSide\",\"uuid\":\"178f6c5d-529f-4f0d-80ca-fb6729cf398e\"}]},\"type\":\"ConnectorPlacement.EquallySpacedConnector\",\"uuid\":\"d5293939-72db-46a2-88f3-163e4f70d202\"}],\"packageUris\":[\"http://schema.mathworks.com/mf0/Connector/R2020b\"],\"version\":\"1.0\"}"
  Bus1 : Outport
  Bus2 : Outport  Port=2
  Bus3 : Outport  Port=3
  Bus4 : Outport  Port=4
  Bus5 : Outport  Port=5
  Bus6 : Outport  Port=6
  Bus7 : Outport  Port=7
  Bus8 : Outport  Port=8
  A=B : Outport  Port=9
  A>B : Outport  Port=10
  Overflow : Outport  Port=11
  wires:
  Subsystem8/1(Carry Out) -> Subsystem2/2(Carry In)
  Subsystem6/1(Carry Out) -> Subsystem5/2(Carry In)
  Subsystem3/1(Carry Out) -> Subsystem6/2(Carry In)
  Subsystem8/2(Bus) -> Bus8/1
  Subsystem7/2(Bus) -> Bus1/1
  Subsystem4/2(Bus) -> Bus2/1
  Subsystem5/2(Bus) -> Bus3/1
  Subsystem6/2(Bus) -> Bus4/1
  Subsystem3/2(Bus) -> Bus5/1
  Subsystem1/2(Bus) -> Bus6/1
  Subsystem2/2(Bus) -> Bus7/1
  Subtract mode/1 -> Subsystem8/2(Carry In), Subsystem8/5(Subtract), Subsystem7/5(Subtract), Subsystem2/5(Subtract), Subsystem4/5(Subtract), Subsystem1/5(Subtract), Subsystem5/5(Subtract), Subsystem6/5(Subtract), Subsystem3/5(Subtract)
  Subsystem7/1(Carry Out) -> Overflow/1
  Bus_A/1 -> Delay One Step3/1  "Bus A"
  MATLAB Function1/1(Decimal) -> Display1/1
  Bus_B/1 -> Delay One Step1/1  "Bus B"
  MATLAB Function3/1(Decimal) -> Display3/1
  Subsystem2/1(Carry Out) -> Subsystem1/2(Carry In)
  Subsystem1/1(Carry Out) -> Subsystem3/2(Carry In)
  Subsystem5/1(Carry Out) -> Subsystem4/2(Carry In)
  Subsystem4/1(Carry Out) -> Subsystem7/2(Carry In)
  Neg_A/1 -> Subsystem8/1(Neg_A), Subsystem2/1(Neg_A), Subsystem1/1(Neg_A), Subsystem6/1(Neg_A), Subsystem5/1(Neg_A), Subsystem4/1(Neg_A), Subsystem7/1(Neg_A), Subsystem3/1(Neg_A)
  Delay One Step3/1 -> MATLAB Function1/1(Binary), Demux2/1
  Delay One Step1/1 -> MATLAB Function3/1(Binary), Demux1/1
  Demux1/1 -> Subsystem7/3(B)
  Demux1/2 -> Subsystem4/3(B)
  Demux1/3 -> Subsystem5/3(B)
  Demux1/4 -> Subsystem6/3(B)
  Demux1/5 -> Subsystem3/3(B)
  Demux1/6 -> Subsystem1/3(B)
  Demux1/7 -> Subsystem2/3(B)
  Demux1/8 -> Subsystem8/3(B)
  Demux2/8 -> Subsystem8/4(A)
  Demux2/7 -> Subsystem2/4(A)
  Demux2/6 -> Subsystem1/4(A)
  Demux2/5 -> Subsystem3/4(A)
  Demux2/4 -> Subsystem6/4(A)
  Demux2/3 -> Subsystem5/4(A)
  Demux2/2 -> Subsystem4/4(A)
  Demux2/1 -> Subsystem7/4(A)
  Subsystem7/3(A >B Next) -> Subsystem4/6(A>B Prev)
  Subsystem7/4(= Currently) -> Subsystem4/7(= So far)
  Subsystem4/4(= Currently) -> Subsystem5/7(= So far)
  Subsystem4/3(A >B Next) -> Subsystem5/6(A>B Prev)
  Subsystem5/4(= Currently) -> Subsystem6/7(= So far)
  Subsystem5/3(A >B Next) -> Subsystem6/6(A>B Prev)
  Constant/1 -> Subsystem7/7(= So far)
  Subsystem1/3(= Currently) -> Subsystem2/6(= So far)
  Subsystem1/4(A >B Next) -> Subsystem2/7(A>B Prev)
  Subsystem3/4(A >B Next) -> Subsystem1/7(A>B Prev)
  Subsystem3/3(= Currently) -> Subsystem1/6(= So far)
  Subsystem2/4(A >B Next) -> Subsystem8/7(A>B Prev)
  Subsystem2/3(= Currently) -> Subsystem8/6(= So far)
  Subsystem8/4(A >B Next) -> A>B/1
  Subsystem8/3(= Currently) -> A=B/1
  Subsystem6/4(= Currently) -> Subsystem3/6(= So far)
  Subsystem6/3(A >B Next) -> Subsystem3/7(A>B Prev)
  Constant1/1 -> Subsystem7/6(A>B Prev)

== system DataPath/Subsystem/ALU/FlagAndDecode ==
  note: A/B/C
  SM : Inport
  Sel_A : Inport  Port=2
  Sel_B : Inport  Port=3
  Sel_C : Inport  Port=4
  ALU Bus : Inport  Port=5
  Overflow : Inport  Port=6
  AND1 : Logic  IconShape=distinctive  AllPortsSameDT=off  OutDataTypeStr=boolean
  AND{3..10} (8 alike) : Logic  Inputs=3  IconShape=distinctive  AllPortsSameDT=off  OutDataTypeStr=boolean
  AND2 : Logic  IconShape=distinctive  AllPortsSameDT=off  OutDataTypeStr=boolean
  Demux1 : Demux  Outputs=8
  NAND : Logic  Operator=NAND  IconShape=distinctive  AllPortsSameDT=off  OutDataTypeStr=boolean
  NOR1 : Logic  Operator=NOR  Inputs=8  IconShape=distinctive  AllPortsSameDT=off  OutDataTypeStr=boolean
  NOT{,1..3} (4 alike) : Logic  Operator=NOT  IconShape=distinctive  AllPortsSameDT=off  OutDataTypeStr=boolean
  0/0/0 : Outport
  0/0/1 : Outport  Port=2
  0/1/0 : Outport  Port=3
  0/1/1 : Outport  Port=4
  1/0/0 : Outport  Port=5
  1/0/1 : Outport  Port=6
  1/1/0 : Outport  Port=7
  1/1/1 : Outport  Port=8
  Zero : Outport  Port=9
  Negative : Outport  Port=10
  wires:
  SM/1 -> AND2/1, NOT/1
  Demux1/1 -> NOR1/1, AND2/2
  NOT/1 -> NAND/2
  Demux1/4 -> NOR1/4
  NOR1/1 -> AND1/2  "Byte_zero"
  Overflow/1 -> NAND/1
  Demux1/5 -> NOR1/5
  NAND/1 -> AND1/1  "No_Overflow"
  Demux1/8 -> NOR1/8
  Demux1/6 -> NOR1/6
  ALU Bus/1 -> Demux1/1
  Demux1/7 -> NOR1/7
  Demux1/3 -> NOR1/3
  AND1/1 -> Zero/1  "Zero"
  AND2/1 -> Negative/1
  Demux1/2 -> NOR1/2
  AND3/1 -> 0/0/0/1
  NOT1/1 -> AND6/1, AND5/1, AND4/1, AND3/1
  AND9/1 -> 1/1/0/1
  Sel_C/1 -> AND10/3, AND8/3, AND6/3, AND4/3, NOT3/1
  AND7/1 -> 1/0/0/1
  AND6/1 -> 0/1/1/1
  NOT2/1 -> AND4/2, AND7/2, AND8/2, AND3/2
  Sel_B/1 -> AND10/2, AND9/2, AND6/2, AND5/2, NOT2/1
  AND4/1 -> 0/0/1/1
  NOT3/1 -> AND9/3, AND7/3, AND5/3, AND3/3
  Sel_A/1 -> AND10/1, AND9/1, AND8/1, AND7/1, NOT1/1
  AND5/1 -> 0/1/0/1
  AND8/1 -> 1/0/1/1
  AND10/1 -> 1/1/1/1

== system DataPath/Subsystem/ALU Regs/A1 ==
  Data bus : Inport
  Store : Inport  Port=2
  CLK : Inport  Port=3
  Demux : Demux  Outputs=8
  Mux : Mux  Inputs=8
  Subsystem1 : Subsystem
  Subsystem2 : Subsystem
  Subsystem3 : Subsystem
  Subsystem4 : Subsystem
  Subsystem5 : Subsystem
  Subsystem6 : Subsystem
  Subsystem7 : Subsystem
  Subsystem8 : Subsystem
  "Q Bus " : Outport
  wires:
  Demux/4 -> Subsystem2/1(Data)
  Mux/1 -> "Q Bus "/1
  Demux/2 -> Subsystem1/1(Data)
  Data bus/1 -> Demux/1
  Subsystem6/1(Q) -> Mux/8
  Store/1 -> Subsystem1/2(Store), Subsystem4/2(Store), Subsystem2/2(Store), Subsystem7/2(Store), Subsystem5/2(Store), Subsystem6/2(Store), Subsystem8/2(Store), Subsystem3/2(Store)
  Demux/5 -> Subsystem7/1(Data)
  Demux/7 -> Subsystem8/1(Data)
  Demux/3 -> Subsystem4/1(Data)
  Subsystem7/1(Q) -> Mux/5
  Demux/6 -> Subsystem5/1(Data)
  Subsystem1/1(Q) -> Mux/2
  Demux/1 -> Subsystem3/1(Data)
  Subsystem3/1(Q) -> Mux/1
  Demux/8 -> Subsystem6/1(Data)
  Subsystem8/1(Q) -> Mux/7
  Subsystem2/1(Q) -> Mux/4
  Subsystem4/1(Q) -> Mux/3
  Subsystem5/1(Q) -> Mux/6
  CLK/1 -> Subsystem1/3(Clock), Subsystem4/3(Clock), Subsystem2/3(Clock), Subsystem7/3(Clock), Subsystem5/3(Clock), Subsystem6/3(Clock), Subsystem8/3(Clock), Subsystem3/3(Clock)

== system DataPath/Subsystem/ALU Regs/A2 ==
  Data bus : Inport
  Store : Inport  Port=2
  CLK : Inport  Port=3
  Demux : Demux  Outputs=8
  Mux : Mux  Inputs=8
  Subsystem1 : Subsystem
  Subsystem2 : Subsystem
  Subsystem3 : Subsystem
  Subsystem4 : Subsystem
  Subsystem5 : Subsystem
  Subsystem6 : Subsystem
  Subsystem7 : Subsystem
  Subsystem8 : Subsystem
  "Q Bus " : Outport
  wires:
  Demux/4 -> Subsystem2/1(Data)
  Mux/1 -> "Q Bus "/1
  Demux/2 -> Subsystem1/1(Data)
  Data bus/1 -> Demux/1
  Subsystem6/1(Q) -> Mux/8
  Store/1 -> Subsystem1/2(Store), Subsystem4/2(Store), Subsystem2/2(Store), Subsystem7/2(Store), Subsystem5/2(Store), Subsystem6/2(Store), Subsystem8/2(Store), Subsystem3/2(Store)
  Demux/5 -> Subsystem7/1(Data)
  Demux/7 -> Subsystem8/1(Data)
  Demux/3 -> Subsystem4/1(Data)
  Subsystem7/1(Q) -> Mux/5
  Demux/6 -> Subsystem5/1(Data)
  Subsystem1/1(Q) -> Mux/2
  Demux/1 -> Subsystem3/1(Data)
  Subsystem3/1(Q) -> Mux/1
  Demux/8 -> Subsystem6/1(Data)
  Subsystem8/1(Q) -> Mux/7
  Subsystem2/1(Q) -> Mux/4
  Subsystem4/1(Q) -> Mux/3
  Subsystem5/1(Q) -> Mux/6
  CLK/1 -> Subsystem1/3(Clock), Subsystem4/3(Clock), Subsystem2/3(Clock), Subsystem7/3(Clock), Subsystem5/3(Clock), Subsystem6/3(Clock), Subsystem8/3(Clock), Subsystem3/3(Clock)

== system DataPath/Subsystem/ALU Regs/B1 ==
  Data bus : Inport
  Store : Inport  Port=2
  CLK : Inport  Port=3
  Demux : Demux  Outputs=8
  Mux : Mux  Inputs=8
  Subsystem1 : Subsystem
  Subsystem2 : Subsystem
  Subsystem3 : Subsystem
  Subsystem4 : Subsystem
  Subsystem5 : Subsystem
  Subsystem6 : Subsystem
  Subsystem7 : Subsystem
  Subsystem8 : Subsystem
  "Q Bus " : Outport
  wires:
  Demux/4 -> Subsystem2/1(Data)
  Mux/1 -> "Q Bus "/1
  Demux/2 -> Subsystem1/1(Data)
  Data bus/1 -> Demux/1
  Subsystem6/1(Q) -> Mux/8
  Store/1 -> Subsystem1/2(Store), Subsystem4/2(Store), Subsystem2/2(Store), Subsystem7/2(Store), Subsystem5/2(Store), Subsystem6/2(Store), Subsystem8/2(Store), Subsystem3/2(Store)
  Demux/5 -> Subsystem7/1(Data)
  Demux/7 -> Subsystem8/1(Data)
  Demux/3 -> Subsystem4/1(Data)
  Subsystem7/1(Q) -> Mux/5
  Demux/6 -> Subsystem5/1(Data)
  Subsystem1/1(Q) -> Mux/2
  Demux/1 -> Subsystem3/1(Data)
  Subsystem3/1(Q) -> Mux/1
  Demux/8 -> Subsystem6/1(Data)
  Subsystem8/1(Q) -> Mux/7
  Subsystem2/1(Q) -> Mux/4
  Subsystem4/1(Q) -> Mux/3
  Subsystem5/1(Q) -> Mux/6
  CLK/1 -> Subsystem1/3(Clock), Subsystem4/3(Clock), Subsystem2/3(Clock), Subsystem7/3(Clock), Subsystem5/3(Clock), Subsystem6/3(Clock), Subsystem8/3(Clock), Subsystem3/3(Clock)

== system DataPath/Subsystem/ALU Regs/B2 ==
  Data bus : Inport
  Store : Inport  Port=2
  CLK : Inport  Port=3
  Demux : Demux  Outputs=8
  Mux : Mux  Inputs=8
  Subsystem1 : Subsystem
  Subsystem2 : Subsystem
  Subsystem3 : Subsystem
  Subsystem4 : Subsystem
  Subsystem5 : Subsystem
  Subsystem6 : Subsystem
  Subsystem7 : Subsystem
  Subsystem8 : Subsystem
  "Q Bus " : Outport
  wires:
  Demux/4 -> Subsystem2/1(Data)
  Mux/1 -> "Q Bus "/1
  Demux/2 -> Subsystem1/1(Data)
  Data bus/1 -> Demux/1
  Subsystem6/1(Q) -> Mux/8
  Store/1 -> Subsystem1/2(Store), Subsystem4/2(Store), Subsystem2/2(Store), Subsystem7/2(Store), Subsystem5/2(Store), Subsystem6/2(Store), Subsystem8/2(Store), Subsystem3/2(Store)
  Demux/5 -> Subsystem7/1(Data)
  Demux/7 -> Subsystem8/1(Data)
  Demux/3 -> Subsystem4/1(Data)
  Subsystem7/1(Q) -> Mux/5
  Demux/6 -> Subsystem5/1(Data)
  Subsystem1/1(Q) -> Mux/2
  Demux/1 -> Subsystem3/1(Data)
  Subsystem3/1(Q) -> Mux/1
  Demux/8 -> Subsystem6/1(Data)
  Subsystem8/1(Q) -> Mux/7
  Subsystem2/1(Q) -> Mux/4
  Subsystem4/1(Q) -> Mux/3
  Subsystem5/1(Q) -> Mux/6
  CLK/1 -> Subsystem1/3(Clock), Subsystem4/3(Clock), Subsystem2/3(Clock), Subsystem7/3(Clock), Subsystem5/3(Clock), Subsystem6/3(Clock), Subsystem8/3(Clock), Subsystem3/3(Clock)

== system DataPath/Subsystem/ALU Regs/Subsystem2 ==
  Bus B1 : Inport
  B1 : Inport  Port=2
  B2 : Inport  Port=3
  Bus B 2 : Inport  Port=4
  Demux : Demux  Outputs=8
  Demux1 : Demux  Outputs=8
  MATLAB Function : MATLAB Function  TreatAsAtomicUnit=on
  Multiport Switch{,1..7} (8 alike) : MultiPortSwitch  DataPortOrder=Specify indices  Inputs=2  DataPortIndices={0,1,-1}  SaturateOnIntegerOverflow=off  InputSameDT=off
  Mux : Mux  Inputs=8
  Zero{,1..7} (8 alike) : Constant  Value=0  OutDataTypeStr=Inherit: Inherit via back propagation
  But Out : Outport
  wires:
  Demux1/7 -> Multiport Switch6/3
  Multiport Switch2/1 -> Mux/3
  Demux/4 -> Multiport Switch3/2
  Bus B 2/1 -> Demux1/1
  Multiport Switch6/1 -> Mux/7
  Demux1/1 -> Multiport Switch/3
  Multiport Switch3/1 -> Mux/4
  Zero/1 -> Multiport Switch/4
  MATLAB Function/1(Select) -> Multiport Switch7/1, Multiport Switch6/1, Multiport Switch5/1, Multiport Switch4/1, Multiport Switch3/1, Multiport Switch2/1, Multiport Switch1/1, Multiport Switch/1
  Demux/2 -> Multiport Switch1/2
  Demux/6 -> Multiport Switch5/2
  Demux/8 -> Multiport Switch7/2
  Multiport Switch/1 -> Mux/1
  Demux1/3 -> Multiport Switch2/3
  Zero6/1 -> Multiport Switch6/4
  Bus B1/1 -> Demux/1
  B2/1 -> MATLAB Function/2(A2)
  Zero5/1 -> Multiport Switch5/4
  Zero4/1 -> Multiport Switch4/4
  Demux/5 -> Multiport Switch4/2
  Zero2/1 -> Multiport Switch2/4
  Zero7/1 -> Multiport Switch7/4
  Demux1/4 -> Multiport Switch3/3
  Demux1/5 -> Multiport Switch4/3
  Multiport Switch5/1 -> Mux/6
  Multiport Switch1/1 -> Mux/2
  Demux1/2 -> Multiport Switch1/3
  Mux/1 -> But Out/1
  Zero3/1 -> Multiport Switch3/4
  Zero1/1 -> Multiport Switch1/4
  Demux/7 -> Multiport Switch6/2
  Demux1/8 -> Multiport Switch7/3
  Multiport Switch7/1 -> Mux/8
  Demux1/6 -> Multiport Switch5/3
  Demux/3 -> Multiport Switch2/2
  Multiport Switch4/1 -> Mux/5
  Demux/1 -> Multiport Switch/2
  B1/1 -> MATLAB Function/1(A1)

== system DataPath/Subsystem/ALU Regs/Subsystem4 ==
  Bus A1 : Inport
  A1 : Inport  Port=2
  A2 : Inport  Port=3
  Bus A2 : Inport  Port=4
  Demux : Demux  Outputs=8
  Demux1 : Demux  Outputs=8
  MATLAB Function : MATLAB Function  TreatAsAtomicUnit=on
  Multiport Switch{,1..7} (8 alike) : MultiPortSwitch  DataPortOrder=Specify indices  Inputs=2  DataPortIndices={0,1,-1}  SaturateOnIntegerOverflow=off  InputSameDT=off
  Mux : Mux  Inputs=8
  Zero{,1..7} (8 alike) : Constant  Value=0  OutDataTypeStr=Inherit: Inherit via back propagation
  But Out : Outport
  wires:
  Demux1/7 -> Multiport Switch6/3
  Multiport Switch2/1 -> Mux/3
  Demux/4 -> Multiport Switch3/2
  Bus A2/1 -> Demux1/1
  Multiport Switch6/1 -> Mux/7
  Demux1/1 -> Multiport Switch/3
  Multiport Switch3/1 -> Mux/4
  Zero/1 -> Multiport Switch/4
  MATLAB Function/1(Select) -> Multiport Switch1/1, Multiport Switch7/1, Multiport Switch6/1, Multiport Switch5/1, Multiport Switch4/1, Multiport Switch3/1, Multiport Switch2/1, Multiport Switch/1
  Demux/2 -> Multiport Switch1/2
  Demux/6 -> Multiport Switch5/2
  Demux/8 -> Multiport Switch7/2
  Multiport Switch/1 -> Mux/1
  Demux1/3 -> Multiport Switch2/3
  Zero6/1 -> Multiport Switch6/4
  Bus A1/1 -> Demux/1
  A2/1 -> MATLAB Function/2(A2)
  Zero5/1 -> Multiport Switch5/4
  Zero4/1 -> Multiport Switch4/4
  Demux/5 -> Multiport Switch4/2
  Zero2/1 -> Multiport Switch2/4
  Zero7/1 -> Multiport Switch7/4
  Demux1/4 -> Multiport Switch3/3
  Demux1/5 -> Multiport Switch4/3
  Multiport Switch5/1 -> Mux/6
  Multiport Switch1/1 -> Mux/2
  Demux1/2 -> Multiport Switch1/3
  Mux/1 -> But Out/1
  Zero3/1 -> Multiport Switch3/4
  Zero1/1 -> Multiport Switch1/4
  Demux/7 -> Multiport Switch6/2
  Demux1/8 -> Multiport Switch7/3
  Multiport Switch7/1 -> Mux/8
  Demux1/6 -> Multiport Switch5/3
  Demux/3 -> Multiport Switch2/2
  Multiport Switch4/1 -> Mux/5
  Demux/1 -> Multiport Switch/2
  A1/1 -> MATLAB Function/1(A1)
